simulink model "sim1"  (R2024a)
settings: Solver=FixedStepAuto  StartTime=0.0  StopTime=10.0  FixedStep=0.001  RelTol=1e-3
model workspace (MAT data in the model file):
  x = Simulink.Signal
  x.DataType = 'auto'
  x.Dimensions = -1
  x.DimensionsMode = 'auto'
  x.Complexity = 'auto'
  x.SampleTime = -1
  x.SamplingMode = 'auto'
  xin = Simulink.Signal
  xin.DataType = 'auto'
  xin.Dimensions = -1
  xin.DimensionsMode = 'auto'
  xin.Complexity = 'auto'
  xin.SampleTime = -1
  xin.SamplingMode = 'auto'
  y = Simulink.Signal
  y.DataType = 'auto'
  y.Dimensions = -1
  y.DimensionsMode = 'auto'
  y.Complexity = 'auto'
  y.SampleTime = -1
  y.SamplingMode = 'auto'
  yout = Simulink.Signal
  yout.DataType = 'auto'
  yout.Dimensions = -1
  yout.DimensionsMode = 'auto'
  yout.Complexity = 'auto'
  yout.SampleTime = -1
  yout.SamplingMode = 'auto'
  z = Simulink.Signal
  z.DataType = 'auto'
  z.Dimensions = -1
  z.DimensionsMode = 'auto'
  z.Complexity = 'auto'
  z.SampleTime = -1
  z.SamplingMode = 'auto'
values from neighbouring files (symbols this model uses):
  kgain = 5.0    [sim1.sldd]
settings Model: DataDictionary=sim1.sldd  Creator=18283  LastModifiedBy=18283
settings OptimizationCC: DefaultParameterBehavior=Inlined  EnhancedBackFolding=on  PassReuseOutputArgsAs=Individual arguments  ZeroExternalMemoryAtStartup=off  ZeroInternalMemoryAtStartup=off  OptimizeBlockOrder=speed  DifferentSizesBufferReuse=on  OptimizationCustomize=off  EfficientTunableParamExpr=on
settings DebuggingCC: ParameterTunabilityLossMsg=error
settings SFSimCC: MATLABDynamicMemAlloc=off
settings RTWCC: Description=AUTOSAR  SystemTargetFile=autosar.tlc  GenCodeOnly=on  TemplateMakefile=ert_default_tmf  GenerateReport=on  LaunchReport=on  DataTypeReplacement=CDataTypesFixedWidth  GenerateWebview=on  GenerateCodeMetricsReport=on  CheckMdlBeforeBuild=Warning
settings CodeAppCC: ForceParamTrailComments=on  IgnoreCustomStorageClasses=off  OperatorAnnotations=on  SimulinkDataObjDesc=on  SFDataObjDesc=on  InsertBlockDesc=on
settings STFCustomTargetCC: MultiwordLength=256  ParMdlRefBuildCompliant=on  CompOptLevelCompliant=on  IncludeMdlTerminateFcn=off  CombineOutputUpdateFcns=on  SuppressErrorStatus=on  ERTCustomFileBanners=on  SupportNonFinite=off  SupportComplex=off  SupportContinuousTime=off  SupportNonInlinedSFcns=off  RemoveResetFunc=on  MATLABClassNameForMDSCustomization=Simulink.SoftwareTarget.ERTCustomization  AutosarCompliant=on  GRTInterface=off  LookupTableObjectStructAxisOrder=2,1,3,4,...  LUTObjectStructOrderEvenSpacing=Size,Table,Breakpoints  SystemTargetFile=autosar.tlc
settings ERTTargetCC: TargetLangStandard=C99 (ISO)  ConcurrentExecutionCompliant=off  IncludeMdlTerminateFcn=off  SuppressErrorStatus=on  SupportNonFinite=off  SupportComplex=off  ModelStepFunctionPrototypeControlCompliant=off  CPPClassGenCompliant=off  AutosarCompliant=on  LookupTableObjectStructAxisOrder=2,1,3,4,...  LUTObjectStructOrderEvenSpacing=Size,Table,Breakpoints  InlinedParameterPlacement=NonHierarchical  ERTCustomFileTemplate=example_file_process.tlc  BooleanTrueId=TRUE  BooleanFalseId=FALSE
settings ConfigComp: CovEnable=on  RecordCoverage=on  CovModelRefEnable=on

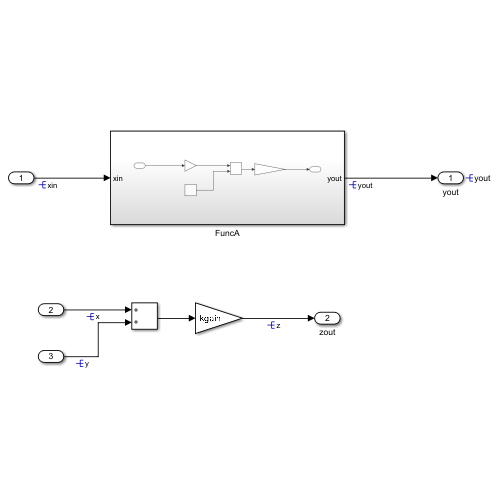
[thumbnail: Simulink's stored preview of the top-level diagram]
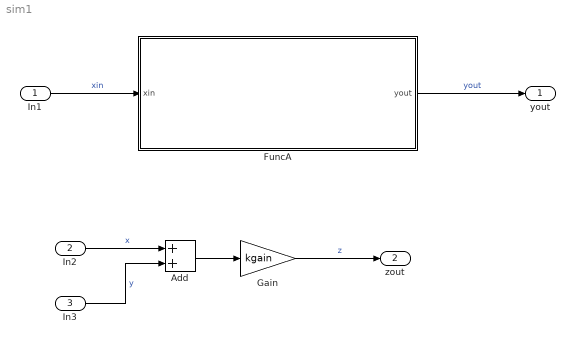
== system sim1 ==
  In1 : Inport
  In2 : Inport  Port=2
  In3 : Inport  Port=3
  Add : Sum
  FuncA : Subsystem
  Gain : Gain  Gain=kgain
  yout : Outport  SignalName=yout
      settings: MustResolveToSignalObject=on
  zout : Outport  Port=2
  wires:
  In1/1 -> FuncA/1(xin)  "xin"
  FuncA/1(yout) -> yout/1  "yout"
  In2/1 -> Add/1  "x"
  In3/1 -> Add/2  "y"
  Add/1 -> Gain/1
  Gain/1 -> zout/1  "z"

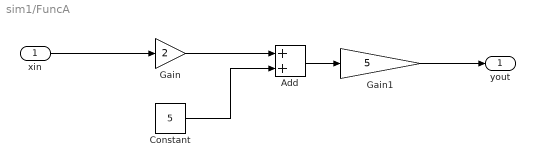
== system sim1/FuncA ==
  xin : Inport
  Add : Sum
  Constant : Constant  Value=5
  Gain : Gain  Gain=2
  Gain1 : Gain  Gain=5
  yout : Outport
  wires:
  Gain/1 -> Add/1
  Gain1/1 -> yout/1
  Constant/1 -> Add/2
  Add/1 -> Gain1/1
  xin/1 -> Gain/1
